simulink model "Simulation_3222"  (R2023a)
settings: Solver=VariableStepAuto  StartTime=0.0  StopTime=600  RelTol=1e-3
undefined symbols (not defined in the file or in its folder): Ion, Lithium
libraries: spsSeriesRLCBranchLib x14, spsBatteryLib x10, spsControlledCurrentSourceLib x10, spsCurrentMeasurementLib x7, spsVoltageMeasurementLib x7, simulink x5, spsControlledVoltageSourceLib x3, spspowerguiLib x1
(part 3 of 3)

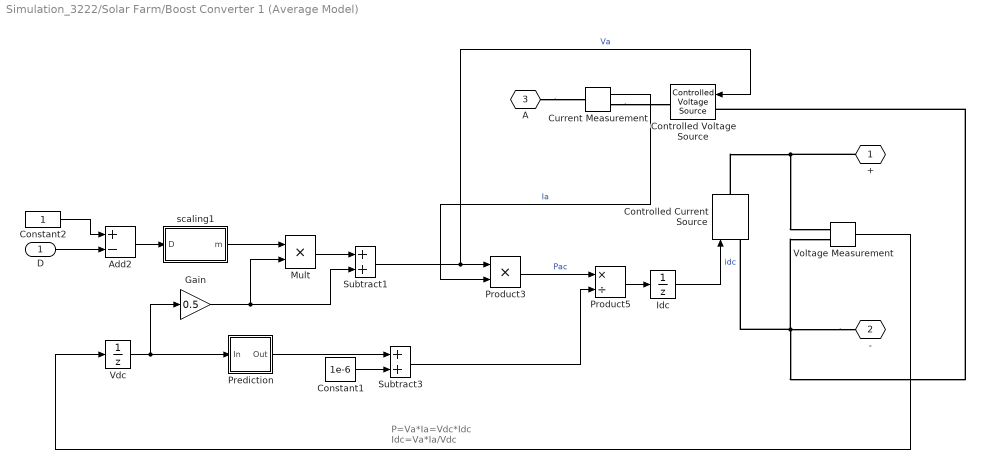
== system Simulation_3222/Solar Farm/Boost Converter 1 (Average Model) ==
  note: P=Va*Ia=Vdc*Idc
      | Idc=Va*Ia/Vdc
  D : Inport
  Add2 : Sum  Inputs=+-
  Constant1 : Constant  Value=1e-6
  Constant2 : Constant
  Controlled Current Source : spsControlledCurrentSourceLib/Controlled Current Source  Initialize=on  Source_Type=AC  Amplitude=0  Phase=0  Frequency=0  Measurements=None
  Controlled Voltage Source : spsControlledVoltageSourceLib/Controlled Voltage Source  Initialize=on  Source_Type=AC  Amplitude=0  Phase=0  Frequency=0  Measurements=None
  Current Measurement : spsCurrentMeasurementLib/Current Measurement  PhasorSimulation=off  OutputType=Complex  PSBequivalent=0
  Gain : Gain  Gain=0.5
  Idc : UnitDelay  SampleTime=Ts  HasFrameUpgradeWarning=on
  Mult : Product  Inputs=**
  Prediction : Subsystem
  Product3 : Product  RndMeth=Zero
  Product5 : Product  Inputs=*/  RndMeth=Zero
  Subtract1 : Sum
  Subtract3 : Sum
  Vdc : UnitDelay  SampleTime=Ts  HasFrameUpgradeWarning=on
  Voltage Measurement : spsVoltageMeasurementLib/Voltage Measurement  PhasorSimulation=off  OutputType=Complex  PSBequivalent=0
  scaling1 : Subsystem
  + : PMIOPort  Tag=PMCPort  Side=Right
  - : PMIOPort  Tag=PMCPort  Port=2  Side=Right
  A : PMIOPort  Tag=PMCPort  Port=3  Side=Left
  wires:
  Gain/1 -> Mult/2, Subtract1/2
  Product5/1 -> Idc/1
  Constant1/1 -> Subtract3/2
  Subtract3/1 -> Product5/2
  Product3/1 -> Product5/1  "Pac"
  Prediction/1(Out) -> Subtract3/1
  Vdc/1 -> Prediction/1(In), Gain/1
  Subtract1/1 -> Product3/1, Controlled Voltage Source/1  "Va"
  Mult/1 -> Subtract1/1
  Constant2/1 -> Add2/1
  Add2/1 -> scaling1/1(D)
  scaling1/1(m) -> Mult/1
  D/1 -> Add2/2
  Voltage Measurement/1 -> Vdc/1
  Idc/1 -> Controlled Current Source/1  "idc"
  Current Measurement/1 -> Product3/2  "Ia"
  connections:
  -/RConn1 -- Voltage Measurement/LConn2 -- Controlled Voltage Source/LConn1 -- Controlled Current Source/LConn1
  +/RConn1 -- Voltage Measurement/LConn1 -- Controlled Current Source/RConn1
  Current Measurement/RConn1 -- Controlled Voltage Source/RConn1
  A/RConn1 -- Current Measurement/LConn1

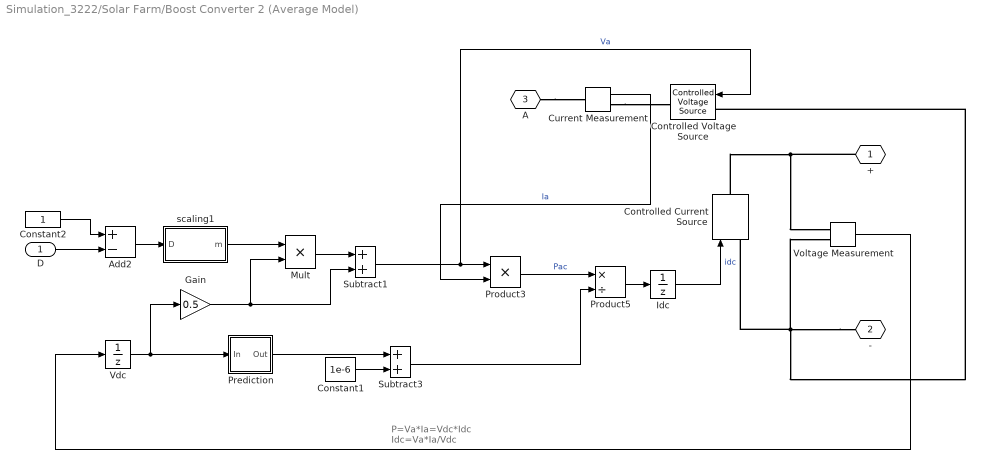
== system Simulation_3222/Solar Farm/Boost Converter 2 (Average Model) ==
  note: P=Va*Ia=Vdc*Idc
      | Idc=Va*Ia/Vdc
  D : Inport
  Add2 : Sum  Inputs=+-
  Constant1 : Constant  Value=1e-6
  Constant2 : Constant
  Controlled Current Source : spsControlledCurrentSourceLib/Controlled Current Source  Initialize=on  Source_Type=AC  Amplitude=0  Phase=0  Frequency=0  Measurements=None
  Controlled Voltage Source : spsControlledVoltageSourceLib/Controlled Voltage Source  Initialize=on  Source_Type=AC  Amplitude=0  Phase=0  Frequency=0  Measurements=None
  Current Measurement : spsCurrentMeasurementLib/Current Measurement  PhasorSimulation=off  OutputType=Complex  PSBequivalent=0
  Gain : Gain  Gain=0.5
  Idc : UnitDelay  SampleTime=Ts  HasFrameUpgradeWarning=on
  Mult : Product  Inputs=**
  Prediction : Subsystem
  Product3 : Product  RndMeth=Zero
  Product5 : Product  Inputs=*/  RndMeth=Zero
  Subtract1 : Sum
  Subtract3 : Sum
  Vdc : UnitDelay  SampleTime=Ts  HasFrameUpgradeWarning=on
  Voltage Measurement : spsVoltageMeasurementLib/Voltage Measurement  PhasorSimulation=off  OutputType=Complex  PSBequivalent=0
  scaling1 : Subsystem
  + : PMIOPort  Tag=PMCPort  Side=Right
  - : PMIOPort  Tag=PMCPort  Port=2  Side=Right
  A : PMIOPort  Tag=PMCPort  Port=3  Side=Left
  wires:
  Gain/1 -> Mult/2, Subtract1/2
  Product5/1 -> Idc/1
  Constant1/1 -> Subtract3/2
  Subtract3/1 -> Product5/2
  Product3/1 -> Product5/1  "Pac"
  Prediction/1(Out) -> Subtract3/1
  Vdc/1 -> Prediction/1(In), Gain/1
  Subtract1/1 -> Product3/1, Controlled Voltage Source/1  "Va"
  Mult/1 -> Subtract1/1
  Constant2/1 -> Add2/1
  Add2/1 -> scaling1/1(D)
  scaling1/1(m) -> Mult/1
  D/1 -> Add2/2
  Voltage Measurement/1 -> Vdc/1
  Idc/1 -> Controlled Current Source/1  "idc"
  Current Measurement/1 -> Product3/2  "Ia"
  connections:
  -/RConn1 -- Voltage Measurement/LConn2 -- Controlled Voltage Source/LConn1 -- Controlled Current Source/LConn1
  +/RConn1 -- Voltage Measurement/LConn1 -- Controlled Current Source/RConn1
  Current Measurement/RConn1 -- Controlled Voltage Source/RConn1
  A/RConn1 -- Current Measurement/LConn1

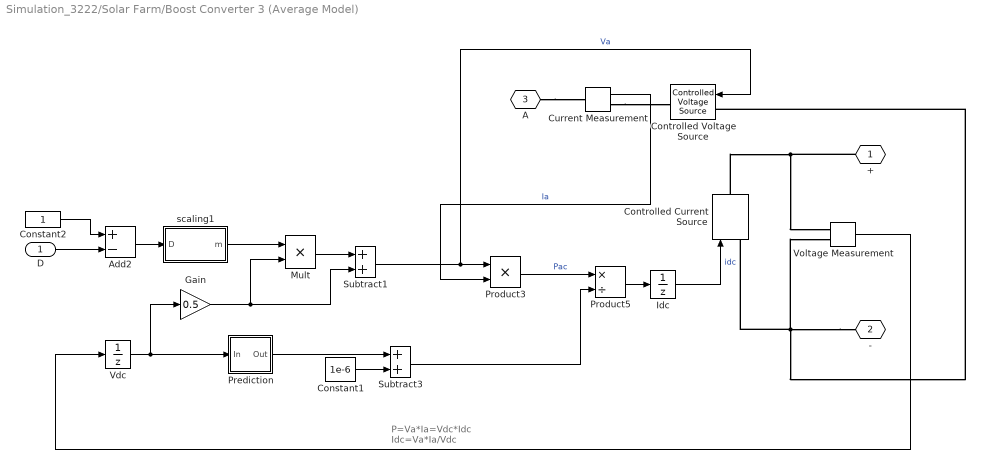
== system Simulation_3222/Solar Farm/Boost Converter 3 (Average Model) ==
  note: P=Va*Ia=Vdc*Idc
      | Idc=Va*Ia/Vdc
  D : Inport
  Add2 : Sum  Inputs=+-
  Constant1 : Constant  Value=1e-6
  Constant2 : Constant
  Controlled Current Source : spsControlledCurrentSourceLib/Controlled Current Source  Initialize=on  Source_Type=AC  Amplitude=0  Phase=0  Frequency=0  Measurements=None
  Controlled Voltage Source : spsControlledVoltageSourceLib/Controlled Voltage Source  Initialize=on  Source_Type=AC  Amplitude=0  Phase=0  Frequency=0  Measurements=None
  Current Measurement : spsCurrentMeasurementLib/Current Measurement  PhasorSimulation=off  OutputType=Complex  PSBequivalent=0
  Gain : Gain  Gain=0.5
  Idc : UnitDelay  SampleTime=Ts  HasFrameUpgradeWarning=on
  Mult : Product  Inputs=**
  Prediction : Subsystem
  Product3 : Product  RndMeth=Zero
  Product5 : Product  Inputs=*/  RndMeth=Zero
  Subtract1 : Sum
  Subtract3 : Sum
  Vdc : UnitDelay  SampleTime=Ts  HasFrameUpgradeWarning=on
  Voltage Measurement : spsVoltageMeasurementLib/Voltage Measurement  PhasorSimulation=off  OutputType=Complex  PSBequivalent=0
  scaling1 : Subsystem
  + : PMIOPort  Tag=PMCPort  Side=Right
  - : PMIOPort  Tag=PMCPort  Port=2  Side=Right
  A : PMIOPort  Tag=PMCPort  Port=3  Side=Left
  wires:
  Gain/1 -> Mult/2, Subtract1/2
  Product5/1 -> Idc/1
  Constant1/1 -> Subtract3/2
  Subtract3/1 -> Product5/2
  Product3/1 -> Product5/1  "Pac"
  Prediction/1(Out) -> Subtract3/1
  Vdc/1 -> Prediction/1(In), Gain/1
  Subtract1/1 -> Product3/1, Controlled Voltage Source/1  "Va"
  Mult/1 -> Subtract1/1
  Constant2/1 -> Add2/1
  Add2/1 -> scaling1/1(D)
  scaling1/1(m) -> Mult/1
  D/1 -> Add2/2
  Voltage Measurement/1 -> Vdc/1
  Idc/1 -> Controlled Current Source/1  "idc"
  Current Measurement/1 -> Product3/2  "Ia"
  connections:
  -/RConn1 -- Voltage Measurement/LConn2 -- Controlled Voltage Source/LConn1 -- Controlled Current Source/LConn1
  +/RConn1 -- Voltage Measurement/LConn1 -- Controlled Current Source/RConn1
  Current Measurement/RConn1 -- Controlled Voltage Source/RConn1
  A/RConn1 -- Current Measurement/LConn1

== system Simulation_3222/Solar Farm/MPPT Parameters ==
  note: Upper limit for D (Dmax)
  note: Increment value used to increase/decrease (DeltaD)
  note: Initial value for D output (Dinit)
  note: (D = Boost converter duty cycle)
  note: Lower limit for D (Dmax)
  note: Parameters for Perturb and Observe Algorithm:
  Iph_ : Constant  Value=0.5
  Iph_1 : Constant  Value=0.52
  Iph_2 : Constant  Value=0.42
  Iph_3 : Constant  Value=3e-4
  Mux : Mux
  Param : Outport
  wires:
  Iph_/1 -> Mux/1
  Iph_1/1 -> Mux/2
  Iph_2/1 -> Mux/3
  Iph_3/1 -> Mux/4
  Mux/1 -> Param/1

== system Simulation_3222/Solar Farm/MPPT Parameters1 ==
  note: Upper limit for D (Dmax)
  note: Increment value used to increase/decrease (DeltaD)
  note: Initial value for D output (Dinit)
  note: (D = Boost converter duty cycle)
  note: Lower limit for D (Dmax)
  note: Parameters for Perturb and Observe Algorithm:
  Iph_ : Constant  Value=0.5
  Iph_1 : Constant  Value=0.52
  Iph_2 : Constant  Value=0.42
  Iph_3 : Constant  Value=3e-4
  Mux : Mux
  Param : Outport
  wires:
  Iph_/1 -> Mux/1
  Iph_1/1 -> Mux/2
  Iph_2/1 -> Mux/3
  Iph_3/1 -> Mux/4
  Mux/1 -> Param/1

== system Simulation_3222/Solar Farm/MPPT Parameters2 ==
  note: Upper limit for D (Dmax)
  note: Increment value used to increase/decrease (DeltaD)
  note: Initial value for D output (Dinit)
  note: (D = Boost converter duty cycle)
  note: Lower limit for D (Dmax)
  note: Parameters for Perturb and Observe Algorithm:
  Iph_ : Constant  Value=0.5
  Iph_1 : Constant  Value=0.52
  Iph_2 : Constant  Value=0.42
  Iph_3 : Constant  Value=3e-4
  Mux : Mux
  Param : Outport
  wires:
  Iph_/1 -> Mux/1
  Iph_1/1 -> Mux/2
  Iph_2/1 -> Mux/3
  Iph_3/1 -> Mux/4
  Mux/1 -> Param/1

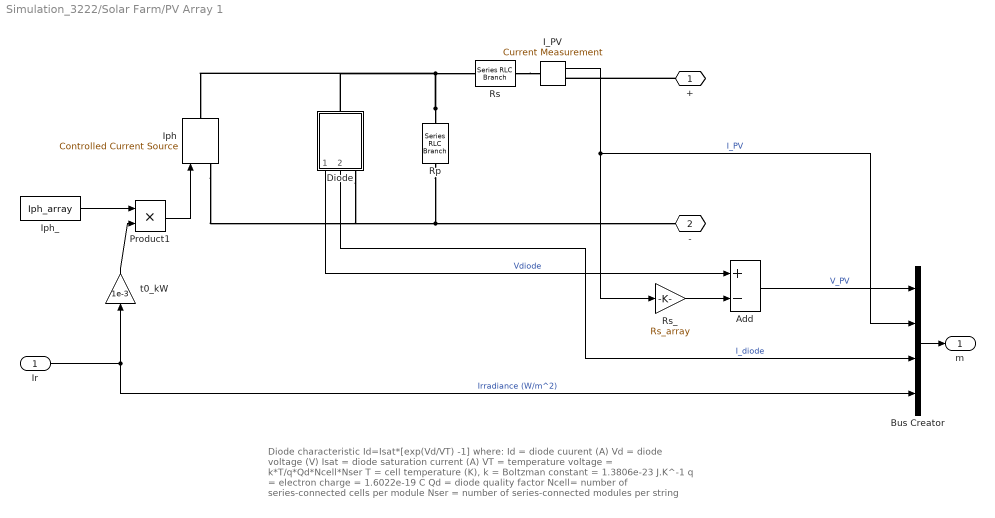
== system Simulation_3222/Solar Farm/PV Array 1 ==
  note: Diode characteristic
      |    Id=Isat*[exp(Vd/VT) -1]
      |
      | where:
      |    Id = diode cuurent (A)
      |    Vd = diode voltage (V)
      |  Isat = diode saturation current (A)
      |    VT = temperature voltage = k*T/q*Qd*Ncell*Nser
      |
      |     T = cell temperature (K),
      |     k = Boltzman constant = 1.3806e-23 J.K^-1
      |     q = electron charge = 1.6022e-19 C
      |    Qd = diode quality factor
      |  Ncell= number of series-connected cells per module
      |  Nser = number of series-connected modules per string
  Ir : Inport
  Add : Sum  Inputs=+-
  Bus Creator : BusCreator  Inputs=4
  Diode : Subsystem
      mask Display:
      | plot(-75,-50,100,150, [-15 -15 43 -15 -15 -75],[50 8 50 92 50 50], ...
      |     [43 43],[8 94],[100 43], [50 50])
  I_PV : spsCurrentMeasurementLib/Current Measurement  PhasorSimulation=off  OutputType=Complex  PSBequivalent=0
  Iph : spsControlledCurrentSourceLib/Controlled Current Source  Initialize=on  Source_Type=AC  Amplitude=0  Phase=0  Frequency=0  Measurements=None
  Iph_ : Constant  Value=Iph_array
  Product1 : Product  Inputs=**  RndMeth=Zero
  Rp : spsSeriesRLCBranchLib/Series RLC Branch  LConnTagsString=__new0  RConnTagsString=__new0  BranchType=R  Resistance=Rp_array  Inductance=1e-3  SetiL0=off  InitialCurrent=0  Capacitance=1e-6  Setx0=off  InitialVoltage=0  Measurements=Branch current
  Rs : spsSeriesRLCBranchLib/Series RLC Branch  LConnTagsString=__new0  RConnTagsString=__new0  BranchType=R  Resistance=Rs_array  Inductance=1e-3  SetiL0=off  InitialCurrent=0  Capacitance=1e-6  Setx0=off  InitialVoltage=0  Measurements=None
  Rs_ : Gain  Gain=Rs_array
  t0_kW : Gain  Gain=1e-3
  + : PMIOPort  Side=Right
  - : PMIOPort  Port=2  Side=Right
  m : Outport
  wires:
  Bus Creator/1 -> m/1
  Diode/2(Idiode) -> Bus Creator/3  "I_diode"
  Add/1 -> Bus Creator/1  "V_PV"
  t0_kW/1 -> Product1/2
  I_PV/1 -> Bus Creator/2, Rs_/1  "I_PV"
  Rs_/1 -> Add/2
  Diode/1(Vdiode) -> Add/1  "Vdiode"
  Ir/1 -> Bus Creator/4, t0_kW/1  "Irradiance (W/m^2)"
  Iph_/1 -> Product1/1
  Product1/1 -> Iph/1
  connections:
  +/RConn1 -- I_PV/RConn1
  Rs/LConn1 -- I_PV/LConn1
  Rp/LConn1 -- Rs/RConn1 -- Iph/RConn1 -- Diode/LConn1
  Rp/RConn1 -- -/RConn1 -- Diode/RConn1 -- Iph/LConn1

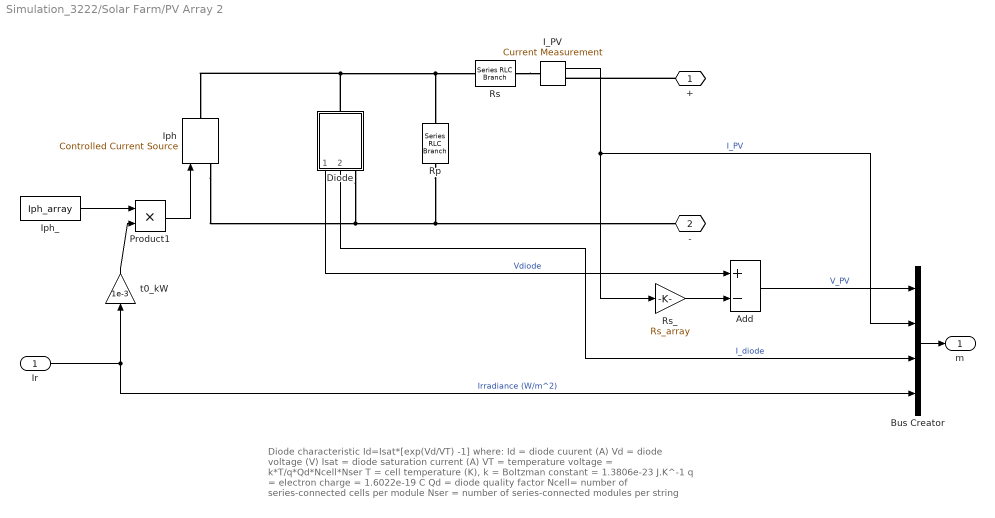
== system Simulation_3222/Solar Farm/PV Array 2 ==
  note: Diode characteristic
      |    Id=Isat*[exp(Vd/VT) -1]
      |
      | where:
      |    Id = diode cuurent (A)
      |    Vd = diode voltage (V)
      |  Isat = diode saturation current (A)
      |    VT = temperature voltage = k*T/q*Qd*Ncell*Nser
      |
      |     T = cell temperature (K),
      |     k = Boltzman constant = 1.3806e-23 J.K^-1
      |     q = electron charge = 1.6022e-19 C
      |    Qd = diode quality factor
      |  Ncell= number of series-connected cells per module
      |  Nser = number of series-connected modules per string
  Ir : Inport
  Add : Sum  Inputs=+-
  Bus Creator : BusCreator  Inputs=4
  Diode : Subsystem
      mask Display:
      | plot(-75,-50,100,150, [-15 -15 43 -15 -15 -75],[50 8 50 92 50 50], ...
      |     [43 43],[8 94],[100 43], [50 50])
  I_PV : spsCurrentMeasurementLib/Current Measurement  PhasorSimulation=off  OutputType=Complex  PSBequivalent=0
  Iph : spsControlledCurrentSourceLib/Controlled Current Source  Initialize=on  Source_Type=AC  Amplitude=0  Phase=0  Frequency=0  Measurements=None
  Iph_ : Constant  Value=Iph_array
  Product1 : Product  Inputs=**  RndMeth=Zero
  Rp : spsSeriesRLCBranchLib/Series RLC Branch  LConnTagsString=__new0  RConnTagsString=__new0  BranchType=R  Resistance=Rp_array  Inductance=1e-3  SetiL0=off  InitialCurrent=0  Capacitance=1e-6  Setx0=off  InitialVoltage=0  Measurements=Branch current
  Rs : spsSeriesRLCBranchLib/Series RLC Branch  LConnTagsString=__new0  RConnTagsString=__new0  BranchType=R  Resistance=Rs_array  Inductance=1e-3  SetiL0=off  InitialCurrent=0  Capacitance=1e-6  Setx0=off  InitialVoltage=0  Measurements=None
  Rs_ : Gain  Gain=Rs_array
  t0_kW : Gain  Gain=1e-3
  + : PMIOPort  Side=Right
  - : PMIOPort  Port=2  Side=Right
  m : Outport
  wires:
  Product1/1 -> Iph/1
  Iph_/1 -> Product1/1
  Ir/1 -> t0_kW/1, Bus Creator/4  "Irradiance (W/m^2)"
  Diode/1(Vdiode) -> Add/1  "Vdiode"
  Rs_/1 -> Add/2
  I_PV/1 -> Rs_/1, Bus Creator/2  "I_PV"
  t0_kW/1 -> Product1/2
  Add/1 -> Bus Creator/1  "V_PV"
  Diode/2(Idiode) -> Bus Creator/3  "I_diode"
  Bus Creator/1 -> m/1
  connections:
  Iph/LConn1 -- Diode/RConn1 -- -/RConn1 -- Rp/RConn1
  Diode/LConn1 -- Iph/RConn1 -- Rs/RConn1 -- Rp/LConn1
  Rs/LConn1 -- I_PV/LConn1
  +/RConn1 -- I_PV/RConn1

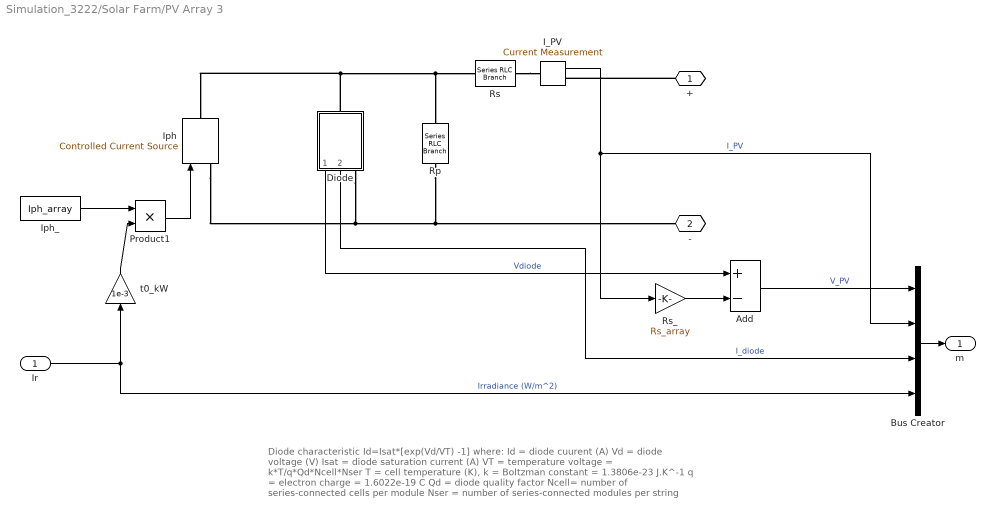
== system Simulation_3222/Solar Farm/PV Array 3 ==
  note: Diode characteristic
      |    Id=Isat*[exp(Vd/VT) -1]
      |
      | where:
      |    Id = diode cuurent (A)
      |    Vd = diode voltage (V)
      |  Isat = diode saturation current (A)
      |    VT = temperature voltage = k*T/q*Qd*Ncell*Nser
      |
      |     T = cell temperature (K),
      |     k = Boltzman constant = 1.3806e-23 J.K^-1
      |     q = electron charge = 1.6022e-19 C
      |    Qd = diode quality factor
      |  Ncell= number of series-connected cells per module
      |  Nser = number of series-connected modules per string
  Ir : Inport
  Add : Sum  Inputs=+-
  Bus Creator : BusCreator  Inputs=4
  Diode : Subsystem
      mask Display:
      | plot(-75,-50,100,150, [-15 -15 43 -15 -15 -75],[50 8 50 92 50 50], ...
      |     [43 43],[8 94],[100 43], [50 50])
  I_PV : spsCurrentMeasurementLib/Current Measurement  PhasorSimulation=off  OutputType=Complex  PSBequivalent=0
  Iph : spsControlledCurrentSourceLib/Controlled Current Source  Initialize=on  Source_Type=AC  Amplitude=0  Phase=0  Frequency=0  Measurements=None
  Iph_ : Constant  Value=Iph_array
  Product1 : Product  Inputs=**  RndMeth=Zero
  Rp : spsSeriesRLCBranchLib/Series RLC Branch  LConnTagsString=__new0  RConnTagsString=__new0  BranchType=R  Resistance=Rp_array  Inductance=1e-3  SetiL0=off  InitialCurrent=0  Capacitance=1e-6  Setx0=off  InitialVoltage=0  Measurements=Branch current
  Rs : spsSeriesRLCBranchLib/Series RLC Branch  LConnTagsString=__new0  RConnTagsString=__new0  BranchType=R  Resistance=Rs_array  Inductance=1e-3  SetiL0=off  InitialCurrent=0  Capacitance=1e-6  Setx0=off  InitialVoltage=0  Measurements=None
  Rs_ : Gain  Gain=Rs_array
  t0_kW : Gain  Gain=1e-3
  + : PMIOPort  Side=Right
  - : PMIOPort  Port=2  Side=Right
  m : Outport
  wires:
  Product1/1 -> Iph/1
  Iph_/1 -> Product1/1
  Ir/1 -> t0_kW/1, Bus Creator/4  "Irradiance (W/m^2)"
  Diode/1(Vdiode) -> Add/1  "Vdiode"
  Rs_/1 -> Add/2
  I_PV/1 -> Rs_/1, Bus Creator/2  "I_PV"
  t0_kW/1 -> Product1/2
  Add/1 -> Bus Creator/1  "V_PV"
  Diode/2(Idiode) -> Bus Creator/3  "I_diode"
  Bus Creator/1 -> m/1
  connections:
  Iph/LConn1 -- Diode/RConn1 -- -/RConn1 -- Rp/RConn1
  Diode/LConn1 -- Iph/RConn1 -- Rs/RConn1 -- Rp/LConn1
  Rs/LConn1 -- I_PV/LConn1
  +/RConn1 -- I_PV/RConn1

== system Simulation_3222/Solar Farm/Subsystem ==
  Repeating Sequence : simulink/Sources/Repeating Sequence  rep_seq_t=[0 479.5 480.5 600]  rep_seq_y=[1361 1020 0 0]
  Out1 : Outport
  wires:
  Repeating Sequence/1 -> Out1/1

== system Simulation_3222/Solar Farm/Boost Converter 1 (Average Model)/Prediction ==
  In : Inport
  Gain : Gain  Gain=2
  Subtract2 : Sum  Inputs=+-
  prediction : UnitDelay  SampleTime=Ts  HasFrameUpgradeWarning=on
  Out : Outport
  wires:
  prediction/1 -> Subtract2/2
  In/1 -> prediction/1, Gain/1
  Subtract2/1 -> Out/1
  Gain/1 -> Subtract2/1

== system Simulation_3222/Solar Farm/Boost Converter 1 (Average Model)/scaling1 ==
  note: Shifting from ]0 to 1[ to a ]-1 to 1[ scale
  D : Inport
  Bias : Bias  Bias=-0.5  SaturateOnIntegerOverflow=off
  Gain : Gain  Gain=2
  Saturation : Saturate  UpperLimit=1  LowerLimit=-1
  m : Outport
  wires:
  Saturation/1 -> m/1
  Gain/1 -> Saturation/1
  D/1 -> Bias/1
  Bias/1 -> Gain/1

== system Simulation_3222/Solar Farm/Boost Converter 2 (Average Model)/Prediction ==
  In : Inport
  Gain : Gain  Gain=2
  Subtract2 : Sum  Inputs=+-
  prediction : UnitDelay  SampleTime=Ts  HasFrameUpgradeWarning=on
  Out : Outport
  wires:
  prediction/1 -> Subtract2/2
  In/1 -> prediction/1, Gain/1
  Subtract2/1 -> Out/1
  Gain/1 -> Subtract2/1

== system Simulation_3222/Solar Farm/Boost Converter 2 (Average Model)/scaling1 ==
  note: Shifting from ]0 to 1[ to a ]-1 to 1[ scale
  D : Inport
  Bias : Bias  Bias=-0.5  SaturateOnIntegerOverflow=off
  Gain : Gain  Gain=2
  Saturation : Saturate  UpperLimit=1  LowerLimit=-1
  m : Outport
  wires:
  Saturation/1 -> m/1
  Gain/1 -> Saturation/1
  D/1 -> Bias/1
  Bias/1 -> Gain/1

== system Simulation_3222/Solar Farm/Boost Converter 3 (Average Model)/Prediction ==
  In : Inport
  Gain : Gain  Gain=2
  Subtract2 : Sum  Inputs=+-
  prediction : UnitDelay  SampleTime=Ts  HasFrameUpgradeWarning=on
  Out : Outport
  wires:
  prediction/1 -> Subtract2/2
  In/1 -> prediction/1, Gain/1
  Subtract2/1 -> Out/1
  Gain/1 -> Subtract2/1

== system Simulation_3222/Solar Farm/Boost Converter 3 (Average Model)/scaling1 ==
  note: Shifting from ]0 to 1[ to a ]-1 to 1[ scale
  D : Inport
  Bias : Bias  Bias=-0.5  SaturateOnIntegerOverflow=off
  Gain : Gain  Gain=2
  Saturation : Saturate  UpperLimit=1  LowerLimit=-1
  m : Outport
  wires:
  Saturation/1 -> m/1
  Gain/1 -> Saturation/1
  D/1 -> Bias/1
  Bias/1 -> Gain/1

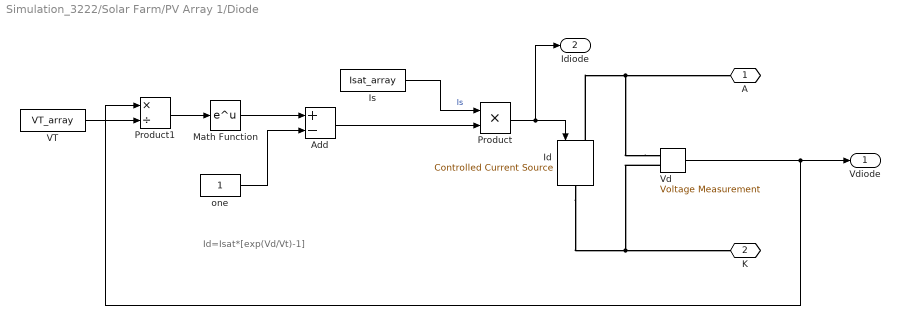
== system Simulation_3222/Solar Farm/PV Array 1/Diode ==
  note: Id=Isat*[exp(Vd/Vt)-1]
  Add : Sum  Inputs=+-
  Id : spsControlledCurrentSourceLib/Controlled Current Source  Initialize=on  Source_Type=AC  Amplitude=0  Phase=0  Frequency=0  Measurements=None
  Is : Constant  Value=Isat_array
  Math Function : Math  SignedPower=on
  Product : Product  RndMeth=Zero
  Product1 : Product  Inputs=*/  RndMeth=Zero
  VT : Constant  Value=VT_array
  Vd : spsVoltageMeasurementLib/Voltage Measurement  PhasorSimulation=off  OutputType=Complex  PSBequivalent=0
  one : Constant
  A : PMIOPort  Side=Left
  K : PMIOPort  Port=2  Side=Right
  Vdiode : Outport
  Idiode : Outport  Port=2
  wires:
  Math Function/1 -> Add/1
  Product/1 -> Idiode/1, Id/1
  Vd/1 -> Product1/1, Vdiode/1
  Is/1 -> Product/1  "Is"
  Product1/1 -> Math Function/1
  one/1 -> Add/2
  Add/1 -> Product/2
  VT/1 -> Product1/2
  connections:
  Id/RConn1 -- K/RConn1 -- Vd/LConn2
  Vd/LConn1 -- A/RConn1 -- Id/LConn1

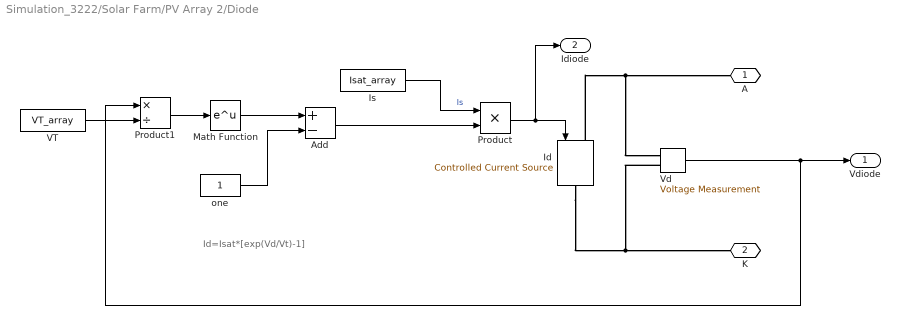
== system Simulation_3222/Solar Farm/PV Array 2/Diode ==
  note: Id=Isat*[exp(Vd/Vt)-1]
  Add : Sum  Inputs=+-
  Id : spsControlledCurrentSourceLib/Controlled Current Source  Initialize=on  Source_Type=AC  Amplitude=0  Phase=0  Frequency=0  Measurements=None
  Is : Constant  Value=Isat_array
  Math Function : Math  SignedPower=on
  Product : Product  RndMeth=Zero
  Product1 : Product  Inputs=*/  RndMeth=Zero
  VT : Constant  Value=VT_array
  Vd : spsVoltageMeasurementLib/Voltage Measurement  PhasorSimulation=off  OutputType=Complex  PSBequivalent=0
  one : Constant
  A : PMIOPort  Side=Left
  K : PMIOPort  Port=2  Side=Right
  Vdiode : Outport
  Idiode : Outport  Port=2
  wires:
  VT/1 -> Product1/2
  Add/1 -> Product/2
  one/1 -> Add/2
  Product1/1 -> Math Function/1
  Is/1 -> Product/1  "Is"
  Vd/1 -> Vdiode/1, Product1/1
  Product/1 -> Id/1, Idiode/1
  Math Function/1 -> Add/1
  connections:
  Id/LConn1 -- A/RConn1 -- Vd/LConn1
  Vd/LConn2 -- K/RConn1 -- Id/RConn1

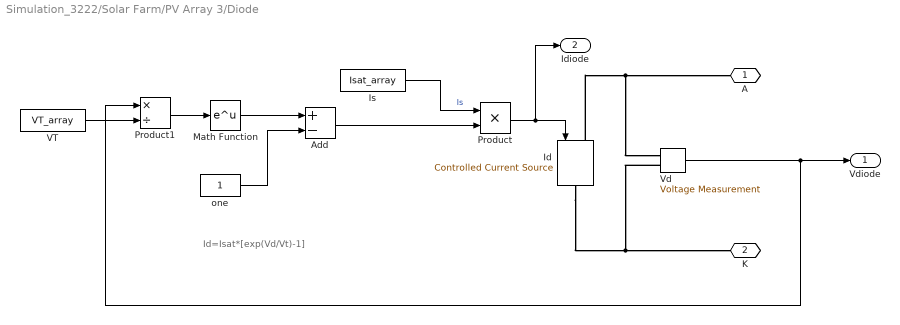
== system Simulation_3222/Solar Farm/PV Array 3/Diode ==
  note: Id=Isat*[exp(Vd/Vt)-1]
  Add : Sum  Inputs=+-
  Id : spsControlledCurrentSourceLib/Controlled Current Source  Initialize=on  Source_Type=AC  Amplitude=0  Phase=0  Frequency=0  Measurements=None
  Is : Constant  Value=Isat_array
  Math Function : Math  SignedPower=on
  Product : Product  RndMeth=Zero
  Product1 : Product  Inputs=*/  RndMeth=Zero
  VT : Constant  Value=VT_array
  Vd : spsVoltageMeasurementLib/Voltage Measurement  PhasorSimulation=off  OutputType=Complex  PSBequivalent=0
  one : Constant
  A : PMIOPort  Side=Left
  K : PMIOPort  Port=2  Side=Right
  Vdiode : Outport
  Idiode : Outport  Port=2
  wires:
  VT/1 -> Product1/2
  Add/1 -> Product/2
  one/1 -> Add/2
  Product1/1 -> Math Function/1
  Is/1 -> Product/1  "Is"
  Vd/1 -> Vdiode/1, Product1/1
  Product/1 -> Id/1, Idiode/1
  Math Function/1 -> Add/1
  connections:
  Id/LConn1 -- A/RConn1 -- Vd/LConn1
  Vd/LConn2 -- K/RConn1 -- Id/RConn1

== matlab function Simulation_3222/Solar Farm/MPPT Controller 3 ==
  settings: updateMethod=DISCRETE  sampleTime=Ts_Control
  data: Param input; Enabled input; V input =V; I input; D output
function D  = PandO(Param, Enabled, V, I)

% MPPT controller based on the Perturb & Observe algorithm.

% D output = Duty cycle of the boost converter (value between 0 and 1)
%
% Enabled input = 1 to enable the MPPT controller
% V input = PV array terminal voltage (V)
% I input = PV array current (A)
%
% Param input:
Dinit = Param(1);  %Initial value for D output
Dmax = Param(2);   %Maximum value for D
Dmin = Param(3);   %Minimum value for D
deltaD = Param(4); %Increment value used to increase/decrease the duty cycle D
% ( increasing D = decreasing Vref )
%  

persistent Vold Pold Dold;

dataType = 'double';

if isempty(Vold)
    Vold=0;
    Pold=0;
    Dold=Dinit;
end
P= V*I;
dV= V - Vold;
dP= P - Pold;

if dP ~= 0 & Enabled ~=0
    if dP < 0
        if dV < 0
            D = Dold - deltaD;
        else
            D = Dold + deltaD;
        end
    else
        if dV < 0
            D = Dold + deltaD;
        else
            D = Dold - deltaD;
        end    
    end
else D=Dold;
end

if D >= Dmax | D<= Dmin
    D=Dold;
end

Dold=D;
Vold=V;
Pold=P;

== matlab function Simulation_3222/Solar Farm/MPPT Controller 1  ==
  settings: updateMethod=DISCRETE  sampleTime=Ts_Control
  data: Param input; Enabled input; V input =V; I input; D output
function D  = PandO(Param, Enabled, V, I)

% MPPT controller based on the Perturb & Observe algorithm.

% D output = Duty cycle of the boost converter (value between 0 and 1)
%
% Enabled input = 1 to enable the MPPT controller
% V input = PV array terminal voltage (V)
% I input = PV array current (A)
%
% Param input:
Dinit = Param(1);  %Initial value for D output
Dmax = Param(2);   %Maximum value for D
Dmin = Param(3);   %Minimum value for D
deltaD = Param(4); %Increment value used to increase/decrease the duty cycle D
% ( increasing D = decreasing Vref )
%  

persistent Vold Pold Dold;

dataType = 'double';

if isempty(Vold)
    Vold=0;
    Pold=0;
    Dold=Dinit;
end
P= V*I;
dV= V - Vold;
dP= P - Pold;

if dP ~= 0 & Enabled ~=0
    if dP < 0
        if dV < 0
            D = Dold - deltaD;
        else
            D = Dold + deltaD;
        end
    else
        if dV < 0
            D = Dold + deltaD;
        else
            D = Dold - deltaD;
        end    
    end
else D=Dold;
end

if D >= Dmax | D<= Dmin
    D=Dold;
end

Dold=D;
Vold=V;
Pold=P;

== matlab function Simulation_3222/Solar Farm/MPPT Controller 2 ==
  settings: updateMethod=DISCRETE  sampleTime=Ts_Control
  data: Param input; Enabled input; V input =V; I input; D output
function D  = PandO(Param, Enabled, V, I)

% MPPT controller based on the Perturb & Observe algorithm.

% D output = Duty cycle of the boost converter (value between 0 and 1)
%
% Enabled input = 1 to enable the MPPT controller
% V input = PV array terminal voltage (V)
% I input = PV array current (A)
%
% Param input:
Dinit = Param(1);  %Initial value for D output
Dmax = Param(2);   %Maximum value for D
Dmin = Param(3);   %Minimum value for D
deltaD = Param(4); %Increment value used to increase/decrease the duty cycle D
% ( increasing D = decreasing Vref )
%  

persistent Vold Pold Dold;

dataType = 'double';

if isempty(Vold)
    Vold=0;
    Pold=0;
    Dold=Dinit;
end
P= V*I;
dV= V - Vold;
dP= P - Pold;

if dP ~= 0 & Enabled ~=0
    if dP < 0
        if dV < 0
            D = Dold - deltaD;
        else
            D = Dold + deltaD;
        end
    else
        if dV < 0
            D = Dold + deltaD;
        else
            D = Dold - deltaD;
        end    
    end
else D=Dold;
end

if D >= Dmax | D<= Dmin
    D=Dold;
end

Dold=D;
Vold=V;
Pold=P;
